simulink model "controllerSharedMemFast"  (Simulink 7.7)
settings: Solver=FixedStepDiscrete  StartTime=0.0  StopTime=inf  FixedStep=1  RelTol=1e-3
InitFcn:
  | initSharedMem;
values from neighbouring files (symbols this model uses):
  k_com = [ 25    0   0]    [initSharedMem.m]
  k_pst = [ diag([k_pst_torso k_pst_arm k_pst_arm k_pst_leg k_pst_leg])    0*eye(25)   0*eye(25)]    [initPartialForceControl.m]    (also in initSharedMem.m)
  kw = 10    [initSharedMem.m]
  nc = 6    [initPartialForceControl.m]    (also in initSharedMem.m = 12)
  nj = 25    [initMonitor.m]    (also in initPartialForceControl.m; initSharedMem.m)
undefined symbols (not defined in the file or in its folder): DiscIntNeverNeededParam
libraries: WBCLibrary x18, simulink x2, dspsigops x2
settings Model: Creator=daniele  LastModifiedBy=daniele
settings DataIOCC: SignalLoggingSaveFormat=Dataset
settings DebuggingCC: FcnCallInpInsideContextMsg=Enable All

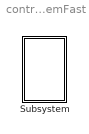
== system controllerSharedMemFast ==
  Subsystem : Subsystem  mask{robotName='icub', Ts=0.01, localName='dynamicBalancing'}
      mask prompts: robotName "robot name"; localName "module name"

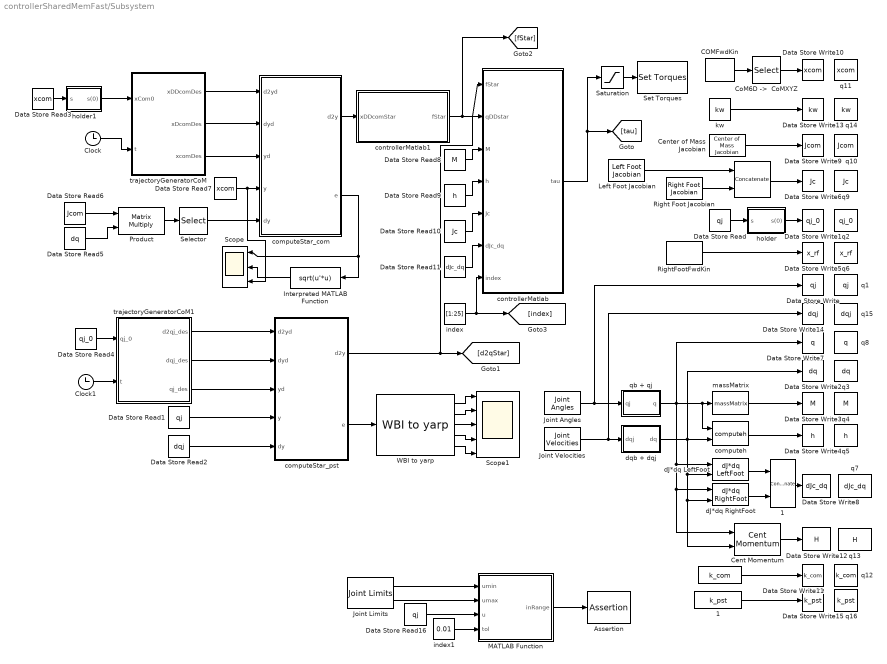
== system controllerSharedMemFast/Subsystem ==
  "    " : Constant  Value=k_com
  "    1" : Constant  Value=k_pst
  " " : Concatenate  Mode=Multidimensional array
  " 1" : Concatenate  Mode=Multidimensional array
  Assertion : Assertion  Enabled=on
  "COMFwdKin " : WBCLibrary/wholeBodyModel/Forward Kinematics/COMFwdKin   robotName=robotName  localName=localName
  Cent Momentum : WBCLibrary/wholeBodyModel/Dynamics/Cent Momentum  robotName=robotName  localName=localName
  Center of Mass Jacobian : WBCLibrary/wholeBodyModel/Jacobians/Center of Mass Jacobian  robotName=robotName  localName=localName
  Clock : Clock
  Clock1 : Clock
  "CoM6D ->  CoMXYZ" : Selector  InputPortWidth=7  IndexOptions=Index vector (dialog)  Indices=[1 2 3]  OutputSizes=1
  Data Store Read : DataStoreRead  DataStoreName=qj
  Data Store Read1 : DataStoreRead  DataStoreName=qj
  Data Store Read10 : DataStoreRead  DataStoreName=Jc
  Data Store Read11 : DataStoreRead  DataStoreName=dJc_dq
  Data Store Read16 : DataStoreRead  DataStoreName=qj
  Data Store Read2 : DataStoreRead  DataStoreName=dqj
  Data Store Read3 : DataStoreRead  DataStoreName=xcom
  Data Store Read4 : DataStoreRead  DataStoreName=qj_0
  Data Store Read5 : DataStoreRead  DataStoreName=dq
  Data Store Read6 : DataStoreRead  DataStoreName=Jcom
  Data Store Read7 : DataStoreRead  DataStoreName=xcom
  Data Store Read8 : DataStoreRead  DataStoreName=M
  Data Store Read9 : DataStoreRead  DataStoreName=h
  Data Store Write : DataStoreWrite  Priority=-1  DataStoreName=qj
  Data Store Write1 : DataStoreWrite  Priority=-1  DataStoreName=qj_0
  Data Store Write10 : DataStoreWrite  Priority=-1  DataStoreName=xcom
  Data Store Write11 : DataStoreWrite  Priority=-1  DataStoreName=k_com
  Data Store Write12 : DataStoreWrite  Priority=-1  DataStoreName=H
  Data Store Write13 : DataStoreWrite  Priority=-1  DataStoreName=kw
  Data Store Write14 : DataStoreWrite  Priority=-1  DataStoreName=dqj
  Data Store Write15 : DataStoreWrite  Priority=-1  DataStoreName=k_pst
  Data Store Write2 : DataStoreWrite  Priority=-1  DataStoreName=dq
  Data Store Write3 : DataStoreWrite  Priority=-1  DataStoreName=M
  Data Store Write4 : DataStoreWrite  Priority=-1  DataStoreName=h
  Data Store Write5 : DataStoreWrite  Priority=-1  DataStoreName=x_rf
  Data Store Write6 : DataStoreWrite  Priority=-1  DataStoreName=Jc
  Data Store Write7 : DataStoreWrite  Priority=-1  DataStoreName=q
  Data Store Write8 : DataStoreWrite  Priority=-1  DataStoreName=dJc_dq
  Data Store Write9 : DataStoreWrite  Priority=-1  DataStoreName=Jcom
  Interpreted MATLAB Function : MATLABFcn  MATLABFcn=sqrt(u'*u)
  Joint Angles : WBCLibrary/wholeBodyStates/Joint Angles  robotName=robotName  localName=localName
  Joint Limits : WBCLibrary/wholeBodyModel/Joint Limits  robotName=robotName  localName=localName
  Joint Velocities : WBCLibrary/wholeBodyStates/Joint Velocities  robotName=robotName  localName=localName
  Left Foot Jacobian : WBCLibrary/wholeBodyModel/Jacobians/Left Foot Jacobian  robotName=robotName  localName=localName
  MATLAB Function : Stateflow chart  TreatAsAtomicUnit=on
      settings: PermitHierarchicalResolution=ParametersOnly
  Product : Product  Multiplication=Matrix(*)  RndMeth=Zero
  Right Foot Jacobian : WBCLibrary/wholeBodyModel/Jacobians/Right Foot Jacobian  robotName=robotName  localName=localName
  RightFootFwdKin : WBCLibrary/wholeBodyModel/Forward Kinematics/RightFootFwdKin  robotName=robotName  localName=localName
  Saturation : Saturate  UpperLimit=12  LowerLimit=-12
  Scope : Scope  NumInputPorts=3
      settings: TimeRange=2500  YMin=-0.03~0.005~-0.075  YMax=0.06~0.065~0.005
  Scope1 : Scope  NumInputPorts=5
      settings: TimeRange=3000  YMin=-0.03~-0.15~-0.2~-0.4~-0.35  YMax=0.015~0.5~0.5~0.1~0.1
  Selector : Selector  InputPortWidth=6  IndexOptions=Index vector (dialog)  Indices=[1:3]  OutputSizes=1
  Set Torques : WBCLibrary/wholeBodyActuators/Set Torques  val=6  robotName=robotName  localName=localName
  WBI to yarp : WBCLibrary/Utilities/WBI to yarp
  computeStar_com : Subsystem  mask{Kp=k_com(1,1).*eye(3), Ki=k_com(1,2).*eye(3), Kd=k_com(1,3).*eye(3)}
  computeStar_pst : Subsystem  mask{Kp=k_pst(1:25,1:25), Kd=k_pst(1:25,26:50), Ki=k_pst(1:25,51:75)}
  computeh : WBCLibrary/wholeBodyModel/Dynamics/computeh  val=7  robotname=robotName  localname=localName
  controllerMatlab : Stateflow chart  TreatAsAtomicUnit=on
      settings: PermitHierarchicalResolution=ParametersOnly
  controllerMatlab1 : Stateflow chart  TreatAsAtomicUnit=on
      settings: PermitHierarchicalResolution=ParametersOnly
  dJ*dq LeftFoot : WBCLibrary/wholeBodyModel/Dynamics/dJ*dq LeftFoot  val=9  robotName=robotName  localName=localName
  dJ*dq RightFoot : WBCLibrary/wholeBodyModel/Dynamics/dJ*dq RightFoot  val=9  robotName=robotName  localName=localName
  dqb + dqj : Subsystem
  holder : Subsystem
  holder1 : Subsystem
  index : Constant  Value=[1:25]  VectorParams1D=off
  index1 : Constant  Value=0.01  VectorParams1D=off
  kw : Constant  Value=kw
  massMatrix : WBCLibrary/wholeBodyModel/Dynamics/massMatrix  val=8  robotname=robotName  localname=localName
  q1 : DataStoreMemory  Priority=-1  DataStoreName=qj  ReadBeforeWriteMsg=warning  WriteAfterWriteMsg=warning  WriteAfterReadMsg=warning  InitialValue=zeros(nj,1)  VectorParams1D=off  OutDataTypeStr=double
  q10 : DataStoreMemory  Priority=-1  DataStoreName=Jcom  ReadBeforeWriteMsg=warning  WriteAfterWriteMsg=warning  WriteAfterReadMsg=warning  InitialValue=zeros(6,nj+6)  VectorParams1D=off  OutDataTypeStr=double
  q11 : DataStoreMemory  Priority=-1  DataStoreName=xcom  ReadBeforeWriteMsg=warning  WriteAfterWriteMsg=warning  WriteAfterReadMsg=warning  InitialValue=zeros(3,1)  VectorParams1D=off  OutDataTypeStr=double
  q12 : DataStoreMemory  Priority=-1  DataStoreName=k_com  ReadBeforeWriteMsg=warning  WriteAfterWriteMsg=warning  WriteAfterReadMsg=warning  InitialValue=k_com  VectorParams1D=off  OutDataTypeStr=double
  q13 : DataStoreMemory  Priority=-1  DataStoreName=H  ReadBeforeWriteMsg=warning  WriteAfterWriteMsg=warning  WriteAfterReadMsg=warning  InitialValue=zeros(6,1)  VectorParams1D=off  OutDataTypeStr=double
  q14 : DataStoreMemory  Priority=-1  DataStoreName=kw  ReadBeforeWriteMsg=warning  WriteAfterWriteMsg=warning  WriteAfterReadMsg=warning  InitialValue=kw  VectorParams1D=off  OutDataTypeStr=double
  q15 : DataStoreMemory  Priority=-1  DataStoreName=dqj  ReadBeforeWriteMsg=warning  WriteAfterWriteMsg=warning  WriteAfterReadMsg=warning  InitialValue=zeros(nj,1)  VectorParams1D=off  OutDataTypeStr=double
  q16 : DataStoreMemory  Priority=-1  DataStoreName=k_pst  ReadBeforeWriteMsg=warning  WriteAfterWriteMsg=warning  WriteAfterReadMsg=warning  InitialValue=k_pst  VectorParams1D=off  OutDataTypeStr=double
  q2 : DataStoreMemory  Priority=-1  DataStoreName=qj_0  ReadBeforeWriteMsg=warning  WriteAfterWriteMsg=warning  WriteAfterReadMsg=warning  InitialValue=zeros(nj,1)  VectorParams1D=off  OutDataTypeStr=double
  q3 : DataStoreMemory  Priority=-1  DataStoreName=dq  ReadBeforeWriteMsg=warning  WriteAfterWriteMsg=warning  WriteAfterReadMsg=warning  InitialValue=zeros(nj+6,1)  VectorParams1D=off  OutDataTypeStr=double
  q4 : DataStoreMemory  Priority=-1  DataStoreName=M  ReadBeforeWriteMsg=warning  WriteAfterWriteMsg=warning  WriteAfterReadMsg=warning  InitialValue=zeros(nj+6,nj+6)  VectorParams1D=off  OutDataTypeStr=double
  q5 : DataStoreMemory  Priority=-1  DataStoreName=h  ReadBeforeWriteMsg=warning  WriteAfterWriteMsg=warning  WriteAfterReadMsg=warning  InitialValue=zeros(nj+6,1)  VectorParams1D=off  OutDataTypeStr=double
  q6 : DataStoreMemory  Priority=-1  DataStoreName=x_rf  ReadBeforeWriteMsg=warning  WriteAfterWriteMsg=warning  WriteAfterReadMsg=warning  InitialValue=zeros(7,1)  VectorParams1D=off  OutDataTypeStr=double
  q7 : DataStoreMemory  Priority=-1  DataStoreName=dJc_dq  ReadBeforeWriteMsg=warning  WriteAfterWriteMsg=warning  WriteAfterReadMsg=warning  InitialValue=zeros(nc,1)  VectorParams1D=off  OutDataTypeStr=double
  q8 : DataStoreMemory  Priority=-1  DataStoreName=q  ReadBeforeWriteMsg=warning  WriteAfterWriteMsg=warning  WriteAfterReadMsg=warning  InitialValue=zeros(nj+16,1)  VectorParams1D=off  OutDataTypeStr=double
  q9 : DataStoreMemory  Priority=-1  DataStoreName=Jc  ReadBeforeWriteMsg=warning  WriteAfterWriteMsg=warning  WriteAfterReadMsg=warning  InitialValue=zeros(nc,nj+6)  VectorParams1D=off  OutDataTypeStr=double
  qb + qj : Subsystem
  trajectoryGeneratorCoM : Stateflow chart  TreatAsAtomicUnit=on
      settings: PermitHierarchicalResolution=ParametersOnly
  trajectoryGeneratorCoM1 : Stateflow chart  TreatAsAtomicUnit=on
      settings: PermitHierarchicalResolution=ParametersOnly
  wires:
  Left Foot Jacobian/1 -> " "/1
  Right Foot Jacobian/1 -> " "/2
  qb + qj/1(q) -> massMatrix/1, computeh/1, dJ*dq LeftFoot/1, dJ*dq RightFoot/1, Cent Momentum/1, Data Store Write7/1
  dqb + dqj/1(dq) -> computeh/2, dJ*dq LeftFoot/2, dJ*dq RightFoot/2, Cent Momentum/2, Data Store Write2/1
  Data Store Read/1 -> holder/1(s)
  holder/1(s(0)) -> Data Store Write1/1
  massMatrix/1 -> Data Store Write3/1
  computeh/1 -> Data Store Write4/1
  Joint Velocities/1 -> dqb + dqj/1(dqj), Data Store Write14/1
  RightFootFwdKin/1 -> Data Store Write5/1
  " "/1 -> Data Store Write6/1
  Center of Mass Jacobian/1 -> Data Store Write9/1
  "COMFwdKin "/1 -> "CoM6D ->  CoMXYZ"/1
  "CoM6D ->  CoMXYZ"/1 -> Data Store Write10/1
  Clock/1 -> trajectoryGeneratorCoM/2(t)
  holder1/1(s(0)) -> trajectoryGeneratorCoM/1(xCom0)
  dJ*dq LeftFoot/1 -> " 1"/1
  dJ*dq RightFoot/1 -> " 1"/2
  " 1"/1 -> Data Store Write8/1
  Cent Momentum/1 -> Data Store Write12/1
  kw/1 -> Data Store Write13/1
  Data Store Read3/1 -> holder1/1(s)
  Clock1/1 -> trajectoryGeneratorCoM1/2(t)
  Data Store Read4/1 -> trajectoryGeneratorCoM1/1(qj_0)
  Joint Angles/1 -> qb + qj/1(qj), Data Store Write/1
  "    "/1 -> Data Store Write11/1
  "    1"/1 -> Data Store Write15/1
  controllerMatlab/1(tau) -> [tau], Saturation/1
  trajectoryGeneratorCoM1/1(d2qj_des) -> computeStar_pst/1(d2yd)
  trajectoryGeneratorCoM1/2(dqj_des) -> computeStar_pst/2(dyd)
  trajectoryGeneratorCoM1/3(qj_des) -> computeStar_pst/3(yd)
  trajectoryGeneratorCoM/1(xDDcomDes) -> computeStar_com/1(d2yd)
  trajectoryGeneratorCoM/2(xDcomDes) -> computeStar_com/2(dyd)
  trajectoryGeneratorCoM/3(xcomDes) -> computeStar_com/3(yd)
  Data Store Read1/1 -> computeStar_pst/4(y)
  Data Store Read2/1 -> computeStar_pst/5(dy)
  Product/1 -> Selector/1
  computeStar_com/1(d2y) -> controllerMatlab1/1(xDDcomStar)
  Data Store Read6/1 -> Product/1
  Data Store Read7/1 -> Scope/3, computeStar_com/4(y)
  Data Store Read5/1 -> Product/2
  Selector/1 -> computeStar_com/5(dy)
  Interpreted MATLAB Function/1 -> Scope/2
  computeStar_com/2(e) -> Interpreted MATLAB Function/1, Scope/1
  controllerMatlab1/1(fStar) -> controllerMatlab/1(fStar), [fStar]
  computeStar_pst/1(d2y) -> controllerMatlab/2(qDDstar), [d2qStar]
  Data Store Read8/1 -> controllerMatlab/3(M)
  Data Store Read9/1 -> controllerMatlab/4(h)
  Data Store Read10/1 -> controllerMatlab/5(Jc)
  Data Store Read11/1 -> controllerMatlab/6(dJc_dq)
  WBI to yarp/1 -> Scope1/1
  WBI to yarp/2 -> Scope1/2
  WBI to yarp/3 -> Scope1/3
  WBI to yarp/4 -> Scope1/4
  WBI to yarp/5 -> Scope1/5
  computeStar_pst/2(e) -> WBI to yarp/1
  index/1 -> [index], controllerMatlab/7(index)
  Joint Limits/1 -> MATLAB Function/1(umin)
  Joint Limits/2 -> MATLAB Function/2(umax)
  Data Store Read16/1 -> MATLAB Function/3(u)
  index1/1 -> MATLAB Function/4(tol)
  MATLAB Function/1(inRange) -> Assertion/1
  Saturation/1 -> Set Torques/1

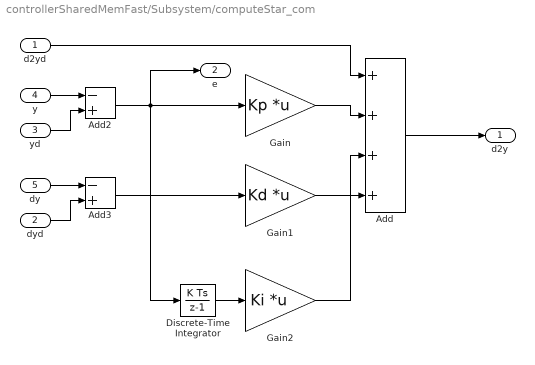
== system controllerSharedMemFast/Subsystem/computeStar_com ==
  d2yd : Inport
  dyd : Inport  Port=2
  yd : Inport  Port=3
  y : Inport  Port=4
  dy : Inport  Port=5
  Add : Sum  Inputs=++++
  Add2 : Sum  Inputs=-+
  Add3 : Sum  Inputs=-+
  Discrete-Time Integrator : DiscreteIntegrator  ICPrevOutput=DiscIntNeverNeededParam  ICPrevScaledInput=DiscIntNeverNeededParam
  Gain : Gain  Gain=Kp  Multiplication=Matrix(K*u)
  Gain1 : Gain  Gain=Kd  Multiplication=Matrix(K*u)
  Gain2 : Gain  Gain=Ki  Multiplication=Matrix(K*u)
  d2y : Outport
  e : Outport  Port=2
  wires:
  Gain/1 -> Add/2
  Gain1/1 -> Add/3
  Gain2/1 -> Add/4
  Add/1 -> d2y/1
  y/1 -> Add2/1
  Add2/1 -> Discrete-Time Integrator/1, Gain/1, e/1
  dy/1 -> Add3/1
  Add3/1 -> Gain1/1
  d2yd/1 -> Add/1
  yd/1 -> Add2/2
  dyd/1 -> Add3/2
  Discrete-Time Integrator/1 -> Gain2/1

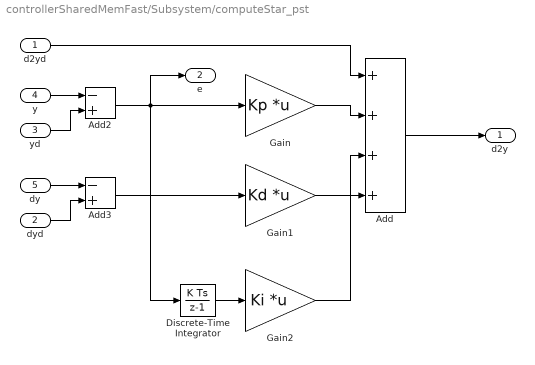
== system controllerSharedMemFast/Subsystem/computeStar_pst ==
  d2yd : Inport
  dyd : Inport  Port=2
  yd : Inport  Port=3
  y : Inport  Port=4
  dy : Inport  Port=5
  Add : Sum  Inputs=++++
  Add2 : Sum  Inputs=-+
  Add3 : Sum  Inputs=-+
  Discrete-Time Integrator : DiscreteIntegrator  ICPrevOutput=DiscIntNeverNeededParam  ICPrevScaledInput=DiscIntNeverNeededParam
  Gain : Gain  Gain=Kp  Multiplication=Matrix(K*u)
  Gain1 : Gain  Gain=Kd  Multiplication=Matrix(K*u)
  Gain2 : Gain  Gain=Ki  Multiplication=Matrix(K*u)
  d2y : Outport
  e : Outport  Port=2
  wires:
  Discrete-Time Integrator/1 -> Gain2/1
  dyd/1 -> Add3/2
  yd/1 -> Add2/2
  d2yd/1 -> Add/1
  Add3/1 -> Gain1/1
  dy/1 -> Add3/1
  Add2/1 -> Discrete-Time Integrator/1, Gain/1, e/1
  y/1 -> Add2/1
  Add/1 -> d2y/1
  Gain2/1 -> Add/4
  Gain1/1 -> Add/3
  Gain/1 -> Add/2

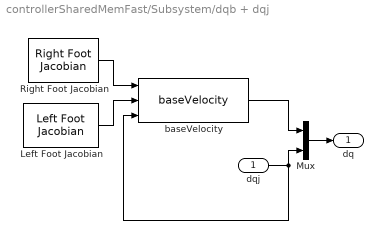
== system controllerSharedMemFast/Subsystem/dqb + dqj ==
  dqj : Inport
  Left Foot Jacobian : WBCLibrary/wholeBodyModel/Jacobians/Left Foot Jacobian  robotName=robotName  localName=localName
  Mux : Mux  Inputs=2
  Right Foot Jacobian : WBCLibrary/wholeBodyModel/Jacobians/Right Foot Jacobian  robotName=robotName  localName=localName
  baseVelocity : WBCLibrary/Utilities/baseVelocity
  dq : Outport
  wires:
  Left Foot Jacobian/1 -> baseVelocity/2
  Right Foot Jacobian/1 -> baseVelocity/1
  baseVelocity/1 -> Mux/1
  dqj/1 -> baseVelocity/3, Mux/2
  Mux/1 -> dq/1

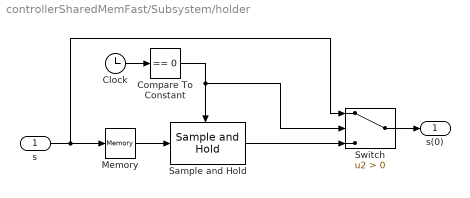
== system controllerSharedMemFast/Subsystem/holder ==
  s : Inport
  Clock : Clock
  Compare To Constant : simulink/Logic and Bit Operations/Compare To Constant  relop===  const=0  LogicOutDataTypeMode=boolean
  Memory : Memory
  Sample and Hold : dspsigops/Sample and Hold  trig=Falling edge  initCond=0  latchinput=off
  Switch : Switch  Criteria=u2 > Threshold
  s(0) : Outport
  wires:
  s/1 -> Switch/1, Memory/1
  Clock/1 -> Compare To Constant/1
  Compare To Constant/1 -> Sample and Hold/Trigger, Switch/2
  Sample and Hold/1 -> Switch/3
  Switch/1 -> s(0)/1
  Memory/1 -> Sample and Hold/1

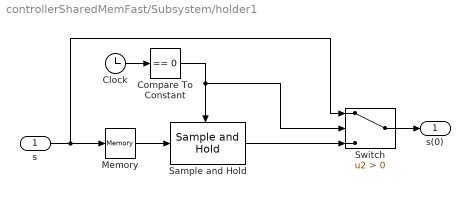
== system controllerSharedMemFast/Subsystem/holder1 ==
  s : Inport
  Clock : Clock
  Compare To Constant : simulink/Logic and Bit Operations/Compare To Constant  relop===  const=0  LogicOutDataTypeMode=boolean
  Memory : Memory
  Sample and Hold : dspsigops/Sample and Hold  trig=Falling edge  initCond=0  latchinput=off
  Switch : Switch  Criteria=u2 > Threshold
  s(0) : Outport
  wires:
  s/1 -> Switch/1, Memory/1
  Clock/1 -> Compare To Constant/1
  Compare To Constant/1 -> Sample and Hold/Trigger, Switch/2
  Sample and Hold/1 -> Switch/3
  Switch/1 -> s(0)/1
  Memory/1 -> Sample and Hold/1

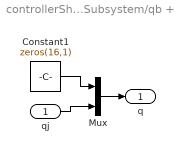
== system controllerSharedMemFast/Subsystem/qb + qj ==
  qj : Inport
  Constant1 : Constant  Value=zeros(16,1)
  Mux : Mux  Inputs=2
  q : Outport
  wires:
  Mux/1 -> q/1
  Constant1/1 -> Mux/1
  qj/1 -> Mux/2

== matlab function Subsystem/trajectoryGeneratorCoM ==
  data: xDDcomDes output double; xDcomDes output double; xcomDes output double; xCom0 input double; t input double; Jcom data_store_memory double; dq data_store_memory double
function [xDDcomDes, xDcomDes, xcomDes]  = trajGen(xCom0,t)
%#codegen


e3 = [0;1;0];
A = 0.05;
f = 0.1;
% t = t*0.8;
% xcomDes    = [xCom0(1:2); (1/A-1)*A*xCom0(3)] + A*xCom0(3)*cos(2*pi*f*t)*e3;
% xDcomDes   = -xCom0(3)*A*2*pi*f*sin(2*pi*f*t)*e3;
% xDDcomDes  = -xCom0(3)*A*(2*pi*f)^2*cos(2*pi*f*t)*e3;

xcomDes    = xCom0 +  A*sin(2*pi*f*t)*e3;
xcomDes(1) =  xcomDes(1) + 0.05;
xDcomDes   =         A*2*pi*f*cos(2*pi*f*t)*e3;
xDDcomDes  =        -A*(2*pi*f)^2*sin(2*pi*f*t)*e3;

== matlab function Subsystem/controllerMatlab ==
  data: fStar input double; qDDstar input double; M input double; h input double; Jc input double; tau output double; dJc_dq input double; index input double
function tau  = computeTau(fStar, qDDstar, M, h, Jc, dJc_dq, index)
%#codegen

PINV_TOL = 1e-5;
g        = 9.81;

Mb    = M(1:6,1:6);
MbInv = inv(Mb);
Mbj   = M(1:6,7:end); 
Mj    = M(7:end,7:end);
U     = [eye(6) , zeros(6,25)];
Jcb   = Jc*U';
SBar  = [  -MbInv*Mbj 
           eye(25)      ];
NjInv = Mj - Mbj'*MbInv*Mbj;

JcSBar     = Jc*SBar;
JcSBarPinv = pinv(JcSBar, PINV_TOL);

% Definition of reference accelerations for CoM and Joints that ensure
% stabilization of desired trajectories xDcomDes and qDes 

Ji     = [zeros(25,6), eye(25)];
Ji     = Ji(index,:);
q_star = qDDstar(index);
% q_star =   -5.*ones(size(q_star));

% We apply the recursion in Del Prete Ph.D. thesis (6.27)
% with N = 2 and d2q_0 = 0. We have:
%
% i = 2 = N
% d2q_2 = JcSBarPinv*(Jcb*MbInv*(h(1:6) - Jcb'*fStar) - dJc_dq);
% N_p2  = I
%
% i = 1
% d2q_1 = d2q_2 + JiSBarN_p1Pinv*(d2x_i - Ji SBar d2q_2)
% N_p1  = N_p2 - pinv(JcSbarN_p2)*JcSbarN_p2

d2q_2 = JcSBarPinv*(Jcb*MbInv*(h(1:6) - Jcb'*fStar) - dJc_dq);
N_p1  = eye(25) - JcSBarPinv * JcSBar;
d2q_1 = d2q_2 + pinv(Ji*SBar*N_p1, PINV_TOL)*(q_star - Ji * SBar * d2q_2);
% d2q_1 = d2q_2;
% tauN  = NjInv*N_p1*d2q_1;

tau = - JcSBar'*fStar + NjInv*d2q_1 + SBar'*[h(1:6);h(7:end)];

== matlab function Subsystem/MATLAB Function ==
  data: umin input double; umax input double; u input double; inRange output double; tol input double
function inRange = checkRange(umin, umax, u, tol)
%#codegen

res = u < umin + tol | u > umax - tol;
res = sum(res);
if res==0
    inRange = 1;
else
    inRange = 0;
    u < umin + tol | u > umax - tol
end

== matlab function Subsystem/trajectoryGeneratorCoM1 ==
  data: d2qj_des output double; dqj_des output double; qj_des output double; qj_0 input double; t input double; Jcom data_store_memory double; dq data_store_memory double
function [d2qj_des, dqj_des, qj_des]  = trajGen(qj_0,t)
%#codegen


qj_des    = qj_0;
dqj_des   = zeros(size(qj_0));
d2qj_des  = zeros(size(qj_0));

== matlab function Subsystem/controllerMatlab1 ==
  data: qj data_store_memory double; qj_0 data_store_memory double; dq data_store_memory double; M data_store_memory double; h data_store_memory double; x_rf data_store_memory double; Jc data_store_memory double; fStar output double; xcom data_store_memory double; xDDcomStar input double; H data_store_memory double; dJc_dq data_store_memory double; kw data_store_memory double
function fStar  = computeF(xDDcomStar)
%#codegen

global M H
global x_rf xcom kw

g        = 9.81;

m     = M(1,1);
grav  = [zeros(2,1);-m*g;zeros(3,1)];

% Definition of reference accelerations for CoM and Joints that ensure
% stabilization of desired trajectories xDcomDes and qDes 


Pr =  x_rf(1:3) - xcom; % Application point of the contact force on the right foot w.r.t. CoM
A  = [ eye(3),   zeros(3),eye(3), zeros(3);
      -Sf(xcom),  eye(3), Sf(Pr), eye(3) ];

% The following expressions for Ic and IcD hold only if the control 
% objective is the stabilization of the CoM's position
% kw = 0.1;
hwDotDes = H(4:end);
hDotDes = [ m*xDDcomStar ;
            -kw*hwDotDes  ]; 

fStar = pinv(A)*(hDotDes-grav);
